simulink model "pi_statelight"  (R2017a)
settings: Solver=VariableStepAuto  StartTime=0.0  StopTime=10.0  RelTol=1e-3
libraries: raspberrypilib x3
settings Model: Creator=Vincent  LastModifiedBy=Vincent

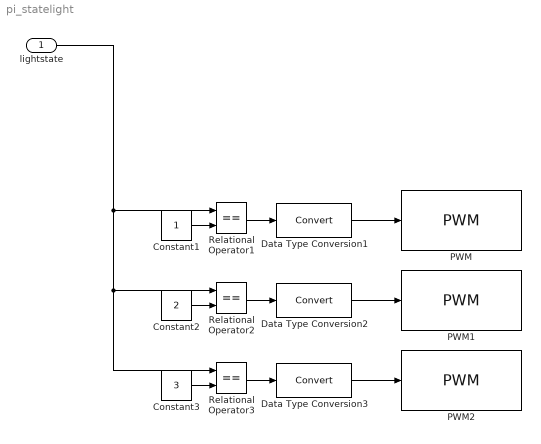
== system pi_statelight ==
  lightstate : Inport
  Constant1 : Constant
  Constant2 : Constant  Value=2
  Constant3 : Constant  Value=3
  Data Type Conversion1 : DataTypeConversion
  Data Type Conversion2 : DataTypeConversion
  Data Type Conversion3 : DataTypeConversion
  PWM : raspberrypilib/PWM  board=Pi 2 Model B  Pin_=21  Frequency=500  blockPlatform=Raspberry Pi
      settings: SourceProductName=Simulink Support Package for Raspberry Pi Hardware  SourceProductBaseCode=RASPPI
  PWM1 : raspberrypilib/PWM  board=Pi 2 Model B  Pin_=26  Frequency=500  blockPlatform=Raspberry Pi
      settings: SourceProductName=Simulink Support Package for Raspberry Pi Hardware  SourceProductBaseCode=RASPPI
  PWM2 : raspberrypilib/PWM  board=Pi 2 Model B  Pin_=20  Frequency=500  blockPlatform=Raspberry Pi
      settings: SourceProductName=Simulink Support Package for Raspberry Pi Hardware  SourceProductBaseCode=RASPPI
  Relational Operator1 : RelationalOperator  Operator===  OutDataTypeStr=boolean  RndMeth=Simplest
  Relational Operator2 : RelationalOperator  Operator===  OutDataTypeStr=boolean  RndMeth=Simplest
  Relational Operator3 : RelationalOperator  Operator===  OutDataTypeStr=boolean  RndMeth=Simplest
  wires:
  Constant2/1 -> Relational Operator2/2
  Relational Operator2/1 -> Data Type Conversion2/1
  Relational Operator3/1 -> Data Type Conversion3/1
  Constant3/1 -> Relational Operator3/2
  Constant1/1 -> Relational Operator1/2
  lightstate/1 -> Relational Operator1/1, Relational Operator2/1, Relational Operator3/1
  Relational Operator1/1 -> Data Type Conversion1/1
  Data Type Conversion1/1 -> PWM/1
  Data Type Conversion2/1 -> PWM1/1
  Data Type Conversion3/1 -> PWM2/1
